simulink model "derpage2"  (R2015b)
settings: Solver=FixedStepDiscrete  SolverMode=SingleTasking  StartTime=0.0  StopTime=63*16  RelTol=1e-3
libraries: dspstat3 x1, dspsigops x1
settings Model: Creator=coltmt  LastModifiedBy=coltmt

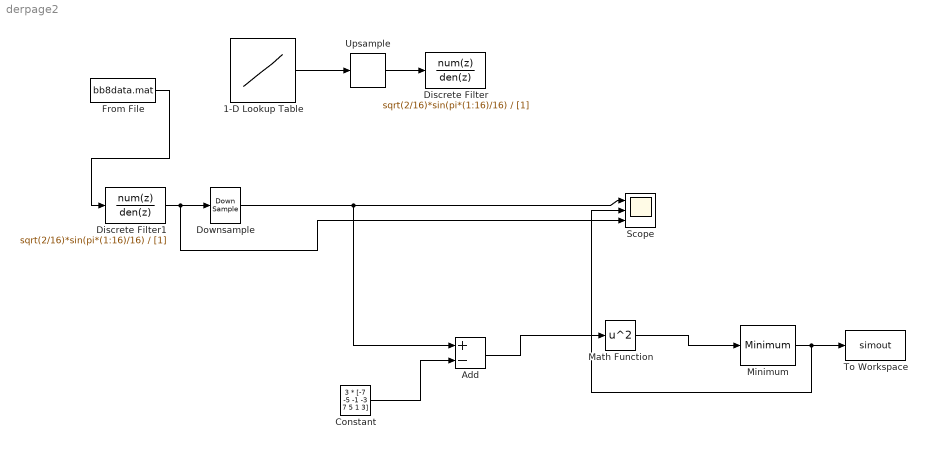
== system derpage2 ==
  1-D Lookup Table : Lookup_n-D  NumberOfTableDimensions=1  BreakpointsForDimension1=[0:7]  Table=3 * [-7 -5 -1 -3 7 5 1 3]  InternalRulePriority=Speed  RndMeth=Simplest  InputSameDT=on
  Add : Sum  Inputs=+-
  Constant : Constant  Value=3 * [-7 -5 -1 -3 7 5 1 3]
  Discrete Filter : DiscreteFilter  Numerator=sqrt(2/16)*sin(pi*(1:16)/16)  Denominator=[1]
  Discrete Filter1 : DiscreteFilter  Numerator=sqrt(2/16)*sin(pi*(1:16)/16)  Denominator=[1]
  Downsample : DownSample  N=16  InputProcessing=Inherited (this choice will be removed - see release notes)  RateOptions=Allow multirate processing
  From File : FromFile  FileName=bb8data.mat  SampleTime=1
  Math Function : Math  Operator=square  SaturateOnIntegerOverflow=on
  Minimum : dspstat3/Minimum  fcn=Index  reset=None  InputProcessing=Columns as channels (frame based)  indexBase=Zero  operateOver=Each column  Dimension=1  operation=minimum  roiEnable=off  roiType=Rectangles  roiPortion=Entire ROI  roiOutput=Individual statistics for each ROI  roiFlag=off  roundingMode=Floor  overflowMode=off
  Scope : Scope  NumInputPorts=3
  To Workspace : ToWorkspace  VariableName=simout  SampleTime=-1
      settings: Save2DSignal=2-D array (concatenate along first dimension)
  Upsample : dspsigops/Upsample  N=16  phase=0  InputProcessing=Inherited (this choice will be removed - see release notes)  RateOptions=Allow multirate processing  ic=0  mode=Unused parameter value
  wires:
  1-D Lookup Table/1 -> Upsample/1
  Upsample/1 -> Discrete Filter/1
  Discrete Filter1/1 -> Scope/3, Downsample/1
  Downsample/1 -> Scope/1, Add/1
  Constant/1 -> Add/2
  Add/1 -> Math Function/1
  Math Function/1 -> Minimum/1
  Minimum/1 -> Scope/2, To Workspace/1
  From File/1 -> Discrete Filter1/1
